simulink library "gbt_library"  (Simulink 7.4)
settings: Solver=ode45  StartTime=0.0  StopTime=10.0  RelTol=1e-3
undefined symbols (not defined in the file or in its folder): xlipgetpartsetting
libraries: xbsIndex_r4 x1348, casper_library_misc x29, casper_library_flow_control x4
(part 1 of 11)
settings Model: Creator=mwagner  LastModifiedBy=chenhong

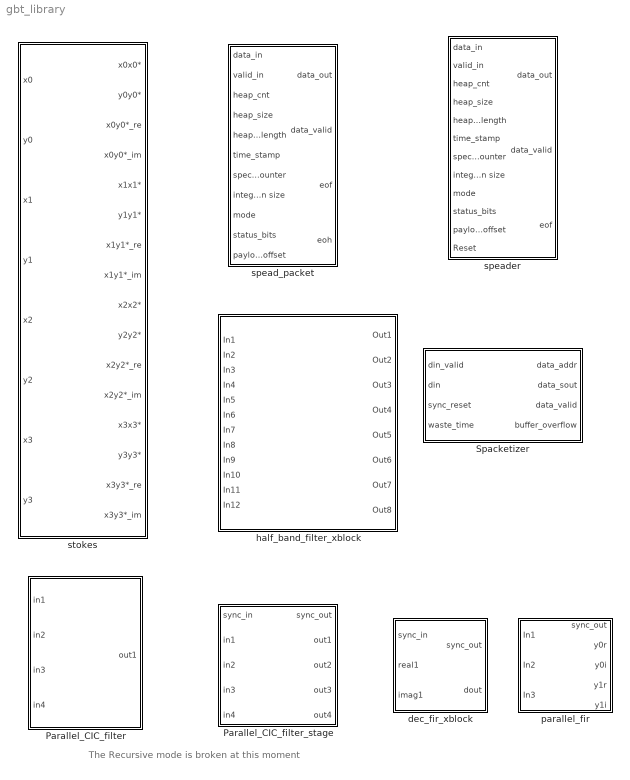
== system gbt_library ==
  note: The Recursive mode is broken at this moment
  Parallel_CIC_filter : Subsystem  mask(Parallel_CIC_filter){m=3, n=100, n_inputs=4, polyphase=off, add_latency=1, n_bits=8, bin_pt=7, dec2_halfout=on, half2first=off, recursive=off}
      mask prompts: m "CIC filter Order"; n "Decimation rate"; polyphase "polyphase structure?(Effective only when n_inputs = 1 or n_inputs = dec_rate)"; add_latency "Add latency"; n_bits "Input bit width"; bin_pt "Binary point"; dec2_halfout "When dec_rate =2, half the number of outputs?"; half2first "Order of stages: Smaller prime factors first?"; recursive "Recursive structure"
      mask help:
      | A non-recursive CIC filter with parallel inputs.
      | Decimation rate is factored into prime numbers. Each implemented using a single stage.
      |
      | For each stages:
      | Only supports decimation rate that is a prime number.
      | If dec_rate = 2, then n_outputs = 0.5*n_inputs.
      | In other cases, n_outputs = n_inputs.
      | Polyphase structure available for stages of n_inputs is 1 or 2.
      mask init:
      | config.source=str2func('parallel_cic_filter_init_xblock');
      | config.toplevel=gcb;
      | set_param(config.toplevel, 'LinkStatus','inactive');
      | xBlock(config, {m,n,n_inputs,...
      |                 polyphase,add_latency,...
      |                 dec2_halfout, half2first,...
      |                 n_bits, bin_pt, recursive} ...
      |                 );
  Parallel_CIC_filter_stage : Subsystem  mask(Parallel_CIC_filter_stage){m=3, n=7, n_inputs=4, polyphase=off, add_latency=1, n_bits=8, bin_pt=7, dec2_halfout=on, recursive=off}
      mask prompts: m "CIC filter Order"; n "Decimation rate"; polyphase "polyphase structure?(Effective only when n_inputs = 1 or n_inputs = dec_rate)"; add_latency "Add latency"; n_bits "Input bit width"; bin_pt "Binary point"; dec2_halfout "When dec_rate =2, half the number of outputs?"; recursive "Recursive structure?"
      mask help:
      | A single stage of CIC filter with parallel inputs.
      | Only supports decimation rate that is a prime number.
      | If dec_rate = 2, then n_outputs = 0.5*n_inputs.
      | In other cases, n_outputs = n_inputs.
      | Polyphase structure available when n_inputs is 1 or 2.
      mask init:
      | xBlock;
      | config.source=str2func('parallel_polynomial_dec_stage_init_xblock');
      | config.toplevel=gcb;
      | xBlock(config, {m,n,n_inputs, ...
      |                 polyphase,add_latency, ...
      |                 dec2_halfout, n_bits, bin_pt,recursive} ...
      |                 );
  Spacketizer : Subsystem  AncestorBlock=gbt_library/packetizer  mask(packetizer){pin_width=256, sout_width=64, fifo_depth=128, total_words=32}
      mask prompts: pin_width "Parallel Input Width"; sout_width "Serial Output Width"; fifo_depth "FIFO depth"; total_words "Total number of data points"
      mask help:
      | This block is intended to serialize data that is 'bursty', that is,
      | the average data rate is small but per cycle the data is highly
      | parallel and can contain many points simultaneously.  This situation
      | is common with the streaming CASPER FFTs and related blocks.
      |
      | The serialization buffers the data when valid and independently
      | serializes the data when the buffer is non-empty.  For convenience, the
      | data is counted as it is serialized and signals exist to indicate
      | that the serial output is valid or that a buffer overflow has occured.  The
      | block will not stop in the case of an overflow, and the overflow
      | signal is not held high after it occurs.
      |
      | For example usage, see 'roach_spec_2adc_borph' in 'SVNROOT/trunk/projects/roach_spec/'
      | or the test case in 'SVNROOT/trunk/mlib_devel_10_1/Tests/packetizer_test.mdl'
      |
      | For extended documentation, please see the CASPER wiki
      mask init:
      | packetizer_init(gcb, 'pin_width', pin_width, 'sout_width', sout_width, 'total_words', total_words, 'fifo_depth', fifo_depth)
      | % packetizer_init(gcb, ...
      | %     'pin_width', pin_width, ...
      | %     'sout_width', sout_width, ...
      | %   %  'fifo_depth', fifo_depth, ...
      | %     'total_words', total_words);
      settings: AttributesFormatString=|
      | Parallel Input Width: 256
      | Serial Output Width: 64
      mask StyleString: edit,edit,popup(16|32|64|128|256|512|1K|2K|4K|8K|16K|32K|64K),edit
  dec_fir_xblock : Subsystem  mask{n_inputs=1, coeff=[0 0], n_bits=4, quantization=Truncate, add_latency=1, mult_latency=2, coeff_bit_width=25, coeff_bin_pt=24, adder_tree_hdl=on}
      mask prompts: n_inputs "Number of Parallel Streams"; coeff "Coefficients"; n_bits "Bit Width Out"; quantization "Quantization Behavior"; add_latency "Add Latency"; mult_latency "Mult Latency"; coeff_bit_width "Coefficient bit width"; coeff_bin_pt "Coefficient binary point"; adder_tree_hdl "Implement first stage of adder trees after multiplication as behavioural HDL"
      mask init:
      | config.source=str2func('dec_fir_init_xblock');
      | config.toplevel=gcb;
      | xBlock(config, ...
      |         {n_inputs,coeff,n_bits,quantization,add_latency,...
      |          mult_latency, coeff_bit_width,coeff_bin_pt,adder_tree_hdl})
      mask StyleString: edit,edit,edit,popup(Truncate|Round  (unbiased: +/- Inf)|Round  (unbiased: Even Values)),edit,edit,edit,edit,checkbox
  half_band_filter_xblock : Subsystem  mask{filter_coeffs=4}
      mask prompts: filter_coeffs "Parallel FIR filter Coefficients"
      mask init:
      | config.source=str2func('half_band_init_xblock');
      | config.toplevel=gcb;
      | xBlock(config, ...
      |         {filter_coeffs})
  parallel_fir : Subsystem  mask(Parallel FIR Filter){filter_coeffs=4}
      mask prompts: filter_coeffs "Filter coefficients"
      mask help: Xblock
      mask init:
      | config.source=str2func('parallel_fir_init_xblock');
      | config.toplevel=gcb;
      | xBlock(config, ...
      |         {filter_coeffs})
  spead_packet : Subsystem  AncestorBlock=gbt_library/spead_packet  mask{spead_msw=64, spead_lsw=40, pkt_bits=6, fifo_latency=4}
      mask help: The size of the heap and payload are in Bytes. If there is one packet per heap then payload_offset is 0. All the input must be not longer than 40 bits.
  speader : Subsystem  AncestorBlock=gbt_library/spead_packet  mask{spead_msw=64, spead_lsw=40, num_items=6}
      mask prompts: num_items "Number of items (+5)"
      mask help:
      | The size of the heap and payload are in Bytes.
      | If there is one packet per heap then payload_offset is 0.
      | All the input must be not longer than 40 bits.
  stokes : Subsystem  mask{n_samples=4}
      mask prompts: n_samples "Number of Simultaneous Inputs"
      mask init:
      | % To make the xBlock smart so it won''t re-generate the
      | % subsystem if neither the arguments nor the scripts are
      | % changes, use as the following:
      | cfg.source = str2func('stokes_init');
      | cfg.toplevel = gcb;
      | cfg.depend = {'stokes_init'};
      | args = {n_samples};
      | xBlock(cfg, args);
      mask TabNameString: Basic

== system gbt_library/Parallel_CIC_filter ==
  in1 : Inport
  in2 : Inport  Port=2
  in3 : Inport  Port=3
  in4 : Inport  Port=4
  Stage1_dec5 : Subsystem
  Stage2_dec5 : Subsystem
  Stage3_dec2 : Subsystem
  Stage4_dec2 : Subsystem
  Terminator{1..4} (4 alike) : Terminator
  out1 : Outport
  wires:
  in1/1 -> Stage4_dec2/1(sync_in), Stage3_dec2/1(sync_in), Stage2_dec5/1(sync_in), Stage1_dec5/2(in1), Stage1_dec5/1(sync_in)
  Stage4_dec2/1(sync_out) -> Terminator4/1  "ter4"
  Stage3_dec2/1(sync_out) -> Terminator3/1  "ter3"
  Stage2_dec5/1(sync_out) -> Terminator2/1  "ter2"
  Stage1_dec5/1(sync_out) -> Terminator1/1  "ter1"
  Stage4_dec2/2(out1) -> out1/1
  Stage3_dec2/3(out2) -> Stage4_dec2/3(in2)  "sig4_2"
  Stage3_dec2/2(out1) -> Stage4_dec2/2(in1)  "sig4_1"
  Stage2_dec5/5(out4) -> Stage3_dec2/5(in4)  "sig3_4"
  Stage2_dec5/4(out3) -> Stage3_dec2/4(in3)  "sig3_3"
  Stage2_dec5/3(out2) -> Stage3_dec2/3(in2)  "sig3_2"
  Stage2_dec5/2(out1) -> Stage3_dec2/2(in1)  "sig3_1"
  Stage1_dec5/5(out4) -> Stage2_dec5/5(in4)  "sig2_4"
  Stage1_dec5/4(out3) -> Stage2_dec5/4(in3)  "sig2_3"
  Stage1_dec5/3(out2) -> Stage2_dec5/3(in2)  "sig2_2"
  Stage1_dec5/2(out1) -> Stage2_dec5/2(in1)  "sig2_1"
  in4/1 -> Stage1_dec5/5(in4)
  in3/1 -> Stage1_dec5/4(in3)
  in2/1 -> Stage1_dec5/3(in2)

== system gbt_library/Parallel_CIC_filter_stage ==
  sync_in : Inport
  in1 : Inport  Port=2
  in2 : Inport  Port=3
  in3 : Inport  Port=4
  in4 : Inport  Port=5
  decimator_7 : Subsystem
  p_adder1 : Subsystem
  p_adder2 : Subsystem
  p_adder3 : Subsystem
  sync_out : Outport
  out1 : Outport  Port=2
  out2 : Outport  Port=3
  out3 : Outport  Port=4
  out4 : Outport  Port=5
  wires:
  decimator_7/5(Out4) -> out4/1
  decimator_7/4(Out3) -> out3/1
  decimator_7/3(Out2) -> out2/1
  decimator_7/2(Out1) -> out1/1
  decimator_7/1(sync_out) -> sync_out/1
  p_adder3/5(out4) -> decimator_7/5(In4)  "pa_i4_4"
  p_adder3/4(out3) -> decimator_7/4(In3)  "pa_i4_3"
  p_adder3/3(out2) -> decimator_7/3(In2)  "pa_i4_2"
  p_adder3/2(out1) -> decimator_7/2(In1)  "pa_i4_1"
  p_adder3/1(sync_out) -> decimator_7/1(sync_in)  "sync_in4"
  p_adder2/5(out4) -> p_adder3/5(in4)  "pa_i3_4"
  p_adder2/4(out3) -> p_adder3/4(in3)  "pa_i3_3"
  p_adder2/3(out2) -> p_adder3/3(in2)  "pa_i3_2"
  p_adder2/2(out1) -> p_adder3/2(in1)  "pa_i3_1"
  p_adder2/1(sync_out) -> p_adder3/1(sync_in)  "sync_in3"
  p_adder1/5(out4) -> p_adder2/5(in4)  "pa_i2_4"
  p_adder1/4(out3) -> p_adder2/4(in3)  "pa_i2_3"
  p_adder1/3(out2) -> p_adder2/3(in2)  "pa_i2_2"
  p_adder1/2(out1) -> p_adder2/2(in1)  "pa_i2_1"
  p_adder1/1(sync_out) -> p_adder2/1(sync_in)  "sync_in2"
  in4/1 -> p_adder1/5(in4)
  in3/1 -> p_adder1/4(in3)
  in2/1 -> p_adder1/3(in2)
  in1/1 -> p_adder1/2(in1)
  sync_in/1 -> p_adder1/1(sync_in)

== system gbt_library/Spacketizer ==
  din_valid : Inport
  din : Inport  Port=2
  sync_reset : Inport  Port=3
  waste_time : Inport  Port=4
  Counter : xbsIndex_r4/Counter  cnt_type=Free Running  cnt_to=Inf  operation=Up  start_count=0  cnt_by_val=1  arith_type=Unsigned  n_bits=11  bin_pt=0  load_pin=off  rst=on  en=on  explicit_period=on  period=1  dbl_ovrd=off  use_behavioral_HDL=off  implementation=Fabric  use_rpm=off  block_type=counter
  Inverter : xbsIndex_r4/Inverter  en=off  latency=0  dbl_ovrd=off  block_type=inv
  Logical : xbsIndex_r4/Logical  logical_function=AND  inputs=2  en=off  latency=0  precision=Full  arith_type=Unsigned  n_bits=16  bin_pt=0  align_bp=on  dbl_ovrd=off  block_type=logical
  Logical1 : xbsIndex_r4/Logical  logical_function=AND  inputs=2  en=off  latency=0  precision=Full  arith_type=Unsigned  n_bits=16  bin_pt=0  align_bp=on  dbl_ovrd=off  block_type=logical
  data_buffer : xbsIndex_r4/FIFO  depth=128  percent_nbits=1  rst=off  en=off  use_dcount=off  use_almost_empty=off  almost_empty_thresh=2  use_almost_full=off  almost_full_thresh=14  dbl_ovrd=off  mem_type=Block RAM  explicit_period=off  block_type=fifo
      settings: block_version=10.1.3
  data_counter : xbsIndex_r4/Counter  cnt_type=Free Running  cnt_to=Inf  operation=Up  start_count=0  cnt_by_val=1  arith_type=Unsigned  n_bits=6  bin_pt=0  load_pin=off  rst=on  en=on  explicit_period=on  period=1  dbl_ovrd=off  use_behavioral_HDL=off  implementation=Fabric  use_rpm=off  block_type=counter
  packetizer_fsm : xbsIndex_r4/MCode  mfname=packetizer_fsm  explicit_period=off  period=1  inputsTable={'boundInpExpr'=>['','','3','','31','','',''],'inputs'=>['fifo_empty','shift_count','data_per_word','data_count','n_words','sync_reset','waste_count','waste_time']}  outputsTable={'outputs'=>['fifo_re','bram_addr_en','bram_we','serializer_shift','serializer_ld','shift_count_en','shift_count_rst','bram_addr_rst','data_count_en','data_count_rst','done','waste_count_en','waste_count_rst'],'suppressOut'=>['off','off','off','off','off','off','off','off','off','off','off','off','off']}  dbl_ovrd=off  enable_stdout=off  enable_debug=off  suppress_output=on  defparams={'data_per_word',3,'n_words',31}  hide_port_list={}  block_type=mcode
      settings: block_version=11.4
  parallel_to_serial_converter : Subsystem  AncestorBlock=casper_library/Flow_Control/parallel_to_serial_converter  mask(parallel_to_serial_converter){pin_width=256, sout_width=64}
      mask prompts: pin_width "Parallel Input Width"; sout_width "Serial Output Width"
      mask help:
      | This block takes as input a parallel bus of specified width.
      | When the load signal 'ld' is asserted, this data is broken into
      | pieces of width specified by the serial output width and
      | stored into different registers chained to form a shift register.
      | If the 'shift' input is subsequently asserted, the shift register
      | returns as output a new piece of data of width sout_width.  This data
      | is the next least significant piece of the original bus.  The converter
      | serializes SMALL ENDIAN.
      |
      | Note that the load operation automatically loads the least significant
      | bits into the register closest to the output, so the first 'shift'
      | assertion changes the data output from bits [sout_width-1:0] to
      | bits [2*sout_width-1:sout_width].
      mask init:
      | parallel_to_serial_converter_init(gcb, ...
      |     'pin_width', pin_width, ...
      |     'sout_width', sout_width);
  shift_counter : xbsIndex_r4/Counter  cnt_type=Free Running  cnt_to=Inf  operation=Up  start_count=0  cnt_by_val=1  arith_type=Unsigned  n_bits=3  bin_pt=0  load_pin=off  rst=on  en=on  explicit_period=on  period=1  dbl_ovrd=off  use_behavioral_HDL=off  implementation=Fabric  use_rpm=off  block_type=counter
  waste_counter : xbsIndex_r4/Counter  cnt_type=Free Running  cnt_to=Inf  operation=Up  start_count=0  cnt_by_val=1  arith_type=Unsigned  n_bits=5  bin_pt=0  load_pin=off  rst=on  en=on  explicit_period=on  period=1  dbl_ovrd=off  use_behavioral_HDL=off  implementation=Fabric  use_rpm=off  block_type=counter
  data_addr : Outport
  data_sout : Outport  Port=2
  data_valid : Outport  Port=3
  buffer_overflow : Outport  Port=4
  wires:
  waste_time/1 -> packetizer_fsm/6
  packetizer_fsm/13 -> waste_counter/1
  packetizer_fsm/12 -> waste_counter/2
  waste_counter/1 -> packetizer_fsm/5
  sync_reset/1 -> packetizer_fsm/4
  packetizer_fsm/10 -> data_counter/1
  data_counter/1 -> packetizer_fsm/3
  packetizer_fsm/9 -> data_counter/2
  packetizer_fsm/8 -> Counter/1
  packetizer_fsm/2 -> Counter/2
  Counter/1 -> data_addr/1
  data_buffer/2 -> packetizer_fsm/1
  packetizer_fsm/7 -> shift_counter/1
  shift_counter/1 -> packetizer_fsm/2
  packetizer_fsm/6 -> shift_counter/2
  parallel_to_serial_converter/1(sout) -> data_sout/1
  din/1 -> data_buffer/1
  packetizer_fsm/3 -> data_valid/1
  packetizer_fsm/5 -> parallel_to_serial_converter/2(ld)
  packetizer_fsm/4 -> parallel_to_serial_converter/3(shift)
  packetizer_fsm/1 -> data_buffer/3
  data_buffer/1 -> parallel_to_serial_converter/1(pin)
  Logical/1 -> data_buffer/2
  din_valid/1 -> Logical/1, Logical1/1
  Inverter/1 -> Logical/2
  data_buffer/4 -> Inverter/1, Logical1/2
  Logical1/1 -> buffer_overflow/1

== system gbt_library/dec_fir_xblock ==
  sync_in : Inport
  real1 : Inport  Port=2
  imag1 : Inport  Port=3
  convert1 : xbsIndex_r4/Convert  arith_type="Signed  (2's comp)"  n_bits=4  bin_pt=3  quantization=Truncate  overflow=Wrap  latency=1  dbl_ovrd=off  pipeline=off  block_type=convert
      settings: block_version=11.4
  convert2 : xbsIndex_r4/Convert  arith_type="Signed  (2's comp)"  n_bits=4  bin_pt=3  quantization=Truncate  overflow=Wrap  latency=1  dbl_ovrd=off  pipeline=off  block_type=convert
      settings: block_version=11.4
  delay : xbsIndex_r4/Delay  en=off  latency=4  dbl_ovrd=off  reg_retiming=off  block_type=delay
      settings: block_version=11.4
  fir_dbl_col1 : Subsystem
  imag_sum : Subsystem
  real_sum : Subsystem
  ri_to_c : casper_library_misc/ri_to_c  SystemSampleTime=-1
  shift1 : xbsIndex_r4/Shift  shift_dir=Left  shift_bits=1  en=off  latency=0  precision=Full  arith_type="Signed  (2's comp)"  n_bits=16  bin_pt=14  quantization=Truncate  overflow=Wrap  dbl_ovrd=off  block_type=shift
  shift2 : xbsIndex_r4/Shift  shift_dir=Left  shift_bits=1  en=off  latency=0  precision=Full  arith_type="Signed  (2's comp)"  n_bits=16  bin_pt=14  quantization=Truncate  overflow=Wrap  dbl_ovrd=off  block_type=shift
  sync_out : Outport
  dout : Outport  Port=2
  wires:
  delay/1 -> real_sum/1(sync), imag_sum/1(sync)
  shift2/1 -> convert2/1
  imag_sum/2(dout) -> shift2/1
  shift1/1 -> convert1/1
  real_sum/2(dout) -> shift1/1
  ri_to_c/1 -> dout/1
  convert2/1 -> ri_to_c/2
  convert1/1 -> ri_to_c/1
  real_sum/1(sync_out) -> sync_out/1
  fir_dbl_col1/5(real_sum) -> real_sum/2(din_1)  "xlsub2_fir_col1_5"
  fir_dbl_col1/6(imag_sum) -> imag_sum/2(din_1)  "xlsub2_fir_col1_6"
  fir_dbl_col1/2(imag_out1) -> fir_dbl_col1/4(imag_back1)  "xlsub2_fir_col1_2"
  fir_dbl_col1/1(real_out1) -> fir_dbl_col1/3(real_back1)  "xlsub2_fir_col1_1"
  imag1/1 -> fir_dbl_col1/2(imag1)
  real1/1 -> fir_dbl_col1/1(real1)
  sync_in/1 -> delay/1

== system gbt_library/half_band_filter_xblock ==
  In1 : Inport
  In2 : Inport  Port=2
  In3 : Inport  Port=3
  In4 : Inport  Port=4
  In5 : Inport  Port=5
  In6 : Inport  Port=6
  In7 : Inport  Port=7
  In8 : Inport  Port=8
  In9 : Inport  Port=9
  In10 : Inport  Port=10
  In11 : Inport  Port=11
  In12 : Inport  Port=12
  adder_tree : Subsystem
  adder_tree1 : Subsystem
  adder_tree3 : Subsystem
  adder_tree4 : Subsystem
  parallel_fir : Subsystem
  parallel_fir1 : Subsystem
  parallel_fir2 : Subsystem
  parallel_fir3 : Subsystem
  Out1 : Outport
  Out2 : Outport  Port=2
  Out3 : Outport  Port=3
  Out4 : Outport  Port=4
  Out5 : Outport  Port=5
  Out6 : Outport  Port=6
  Out7 : Outport  Port=7
  Out8 : Outport  Port=8
  wires:
  parallel_fir3/5(y1i) -> adder_tree4/5(din_4)
  parallel_fir3/4(y1r) -> adder_tree3/5(din_4)
  parallel_fir3/3(y0i) -> adder_tree1/5(din_4)
  parallel_fir3/2(y0r) -> adder_tree/5(din_4)
  parallel_fir3/1(sync_out) -> adder_tree4/1(sync)
  In12/1 -> parallel_fir3/3(In3)
  In11/1 -> parallel_fir3/2(In2)
  In10/1 -> parallel_fir3/1(In1)
  parallel_fir2/5(y1i) -> adder_tree4/4(din_3)
  parallel_fir2/4(y1r) -> adder_tree3/4(din_3)
  parallel_fir2/3(y0i) -> adder_tree1/4(din_3)
  parallel_fir2/2(y0r) -> adder_tree/4(din_3)
  parallel_fir2/1(sync_out) -> adder_tree3/1(sync)
  In9/1 -> parallel_fir2/3(In3)
  In8/1 -> parallel_fir2/2(In2)
  In7/1 -> parallel_fir2/1(In1)
  parallel_fir1/5(y1i) -> adder_tree4/3(din_2)
  parallel_fir1/4(y1r) -> adder_tree3/3(din_2)
  parallel_fir1/3(y0i) -> adder_tree1/3(din_2)
  parallel_fir1/2(y0r) -> adder_tree/3(din_2)
  parallel_fir1/1(sync_out) -> adder_tree1/1(sync)
  In6/1 -> parallel_fir1/3(In3)
  In5/1 -> parallel_fir1/2(In2)
  In4/1 -> parallel_fir1/1(In1)
  parallel_fir/5(y1i) -> adder_tree4/2(din_1)
  parallel_fir/4(y1r) -> adder_tree3/2(din_1)
  parallel_fir/3(y0i) -> adder_tree1/2(din_1)
  parallel_fir/2(y0r) -> adder_tree/2(din_1)
  parallel_fir/1(sync_out) -> adder_tree/1(sync)
  In3/1 -> parallel_fir/3(In3)
  In2/1 -> parallel_fir/2(In2)
  In1/1 -> parallel_fir/1(In1)
  adder_tree4/2(dout) -> Out8/1
  adder_tree4/1(sync_out) -> Out7/1
  adder_tree3/2(dout) -> Out6/1
  adder_tree3/1(sync_out) -> Out5/1
  adder_tree1/2(dout) -> Out4/1
  adder_tree1/1(sync_out) -> Out3/1
  adder_tree/2(dout) -> Out2/1
  adder_tree/1(sync_out) -> Out1/1

== system gbt_library/parallel_fir ==
  In1 : Inport
  In2 : Inport  Port=2
  In3 : Inport  Port=3
  AddSub{1,3,5..6} (4 alike) : xbsIndex_r4/AddSub  mode=Subtraction  use_carryin=off  use_carryout=off  en=off  latency=0  precision=Full  arith_type=Unsigned  n_bits=16  bin_pt=14  quantization=Truncate  overflow=Wrap  dbl_ovrd=off  use_behavioral_HDL=off  hw_selection=Fabric  pipelined=off  block_type=addsub
  AddSub2 : xbsIndex_r4/AddSub  mode=Addition  use_carryin=off  use_carryout=off  en=off  latency=0  precision=Full  arith_type=Unsigned  n_bits=16  bin_pt=14  quantization=Truncate  overflow=Wrap  dbl_ovrd=off  use_behavioral_HDL=off  hw_selection=Fabric  pipelined=off  block_type=addsub
  AddSub4 : xbsIndex_r4/AddSub  mode=Addition  use_carryin=off  use_carryout=off  en=off  latency=0  precision=Full  arith_type=Unsigned  n_bits=16  bin_pt=14  quantization=Truncate  overflow=Wrap  dbl_ovrd=off  use_behavioral_HDL=off  hw_selection=Fabric  pipelined=off  block_type=addsub
  Delay : xbsIndex_r4/Delay  en=off  latency=1  dbl_ovrd=off  reg_retiming=off  block_type=delay
      settings: block_version=11.4
  Delay1 : xbsIndex_r4/Delay  en=off  latency=1  dbl_ovrd=off  reg_retiming=off  block_type=delay
      settings: block_version=11.4
  c_to_ri : Subsystem
  c_to_ri1 : Subsystem
  c_to_ri2 : Subsystem
  f0 : Subsystem
  f0pf1 : Subsystem
  f1 : Subsystem
  sync_out : Outport
  y0r : Outport  Port=2
  y0i : Outport  Port=3
  y1r : Outport  Port=4
  y1i : Outport  Port=5
  wires:
  c_to_ri/1(re) -> AddSub5/1, AddSub2/1
  c_to_ri/2(im) -> AddSub6/1, AddSub4/1
  c_to_ri2/1(re) -> Delay/1, AddSub1/2
  c_to_ri2/2(im) -> Delay1/1, AddSub3/2
  In1/1 -> f1/1(sync_in), f0pf1/1(sync_in), f0/1(sync_in)
  In2/1 -> f1/2(real1), f0pf1/2(real1), f0/2(real1)
  In3/1 -> f1/3(imag1), f0pf1/3(imag1), f0/3(imag1)
  f1/2(dout) -> c_to_ri2/1(c)
  f0pf1/2(dout) -> c_to_ri1/1(c)
  f0/2(dout) -> c_to_ri/1(c)
  f0/1(sync_out) -> sync_out/1
  c_to_ri1/2(im) -> AddSub3/1
  c_to_ri1/1(re) -> AddSub1/1
  Delay1/1 -> AddSub4/2
  Delay/1 -> AddSub2/2
  AddSub6/1 -> y1i/1
  AddSub3/1 -> AddSub6/2
  AddSub5/1 -> y1r/1
  AddSub1/1 -> AddSub5/2
  AddSub4/1 -> y0i/1
  AddSub2/1 -> y0r/1

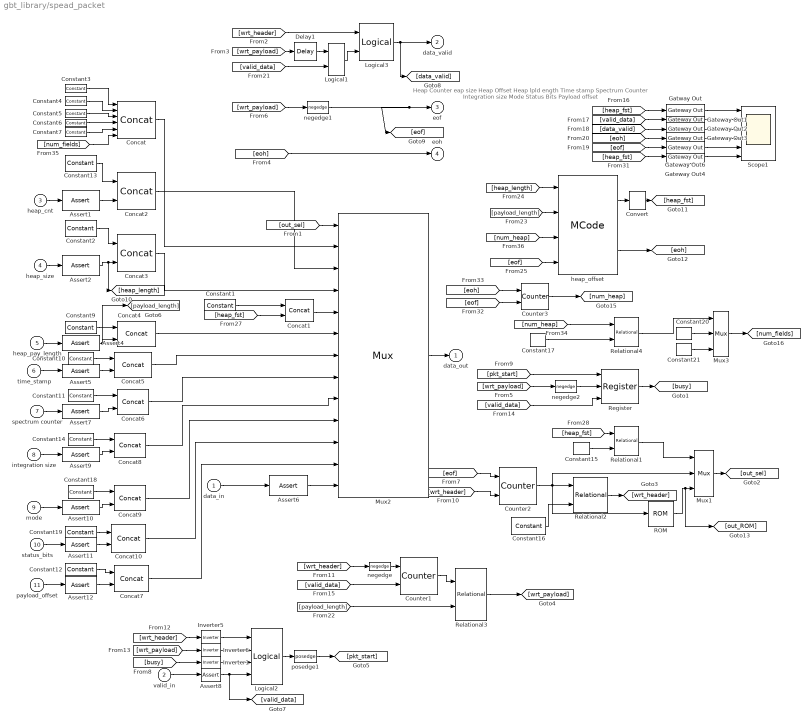
== system gbt_library/spead_packet ==
  note: Heap Counter
      | eap size
      | Heap Offset
      | Heap lpld ength
      | Time stamp
      | Spectrum Counter
      | Integration size
      | Mode
      | Status Bits
      | Payload offset
  data_in : Inport
  valid_in : Inport  Port=2
  heap_cnt : Inport  Port=3
  heap_size : Inport  Port=4
  heap_pay_length : Inport  Port=5
  time_stamp : Inport  Port=6
  spectrum counter : Inport  Port=7
  integration size : Inport  Port=8
  mode : Inport  Port=9
  status_bits : Inport  Port=10
  payload_offset : Inport  Port=11
  Assert{1..2,4..5,7,9..12} (9 alike) : xbsIndex_r4/Assert  assert_type=on  type_source=Explicitly  arith_type=Unsigned  n_bits=spead_lsw  bin_pt=0  assert_rate=off  rate_source=Explicitly  period=1  output_port=on  block_type=assert
      settings: block_version=11.4
  Assert6 : xbsIndex_r4/Assert  assert_type=on  type_source=Explicitly  arith_type=Unsigned  n_bits=64  bin_pt=0  assert_rate=off  rate_source=Explicitly  period=1  output_port=on  block_type=assert
      settings: block_version=11.4
  Assert8 : xbsIndex_r4/Assert  assert_type=on  type_source=Explicitly  arith_type=Boolean  n_bits=64  bin_pt=0  assert_rate=off  rate_source=Explicitly  period=1  output_port=on  block_type=assert
      settings: block_version=11.4
  Concat : xbsIndex_r4/Concat  num_inputs=6  dbl_ovrd=off  block_type=concat
  Concat{1..10} (10 alike) : xbsIndex_r4/Concat  num_inputs=2  dbl_ovrd=off  block_type=concat
  Constant1 : xbsIndex_r4/Constant  arith_type=Unsigned  const=8388611  n_bits=spead_msw-spead_lsw  bin_pt=0  explicit_period=on  period=1  equ=P=C  opselect=C  inp2=PCIN>>17  opr=+  inp1=P  carry=CIN  dbl_ovrd=off  block_type=constant
      settings: block_version=11.4
  Constant10 : xbsIndex_r4/Constant  arith_type=Unsigned  const=8388628  n_bits=spead_msw-spead_lsw  bin_pt=0  explicit_period=on  period=1  equ=P=C  opselect=C  inp2=PCIN>>17  opr=+  inp1=P  carry=CIN  dbl_ovrd=off  block_type=constant
      settings: block_version=11.4
  Constant11 : xbsIndex_r4/Constant  arith_type=Unsigned  const=8388629  n_bits=spead_msw-spead_lsw  bin_pt=0  explicit_period=on  period=1  equ=P=C  opselect=C  inp2=PCIN>>17  opr=+  inp1=P  carry=CIN  dbl_ovrd=off  block_type=constant
      settings: block_version=11.4
  Constant12 : xbsIndex_r4/Constant  arith_type=Unsigned  const=26  n_bits=spead_msw-spead_lsw  bin_pt=0  explicit_period=on  period=1  equ=P=C  opselect=C  inp2=PCIN>>17  opr=+  inp1=P  carry=CIN  dbl_ovrd=off  block_type=constant
      settings: block_version=11.4
  Constant13 : xbsIndex_r4/Constant  arith_type=Unsigned  const=8388609  n_bits=spead_msw-spead_lsw  bin_pt=0  explicit_period=on  period=1  equ=P=C  opselect=C  inp2=PCIN>>17  opr=+  inp1=P  carry=CIN  dbl_ovrd=off  block_type=constant
      settings: block_version=11.4
  Constant14 : xbsIndex_r4/Constant  arith_type=Unsigned  const=8388630  n_bits=spead_msw-spead_lsw  bin_pt=0  explicit_period=on  period=1  equ=P=C  opselect=C  inp2=PCIN>>17  opr=+  inp1=P  carry=CIN  dbl_ovrd=off  block_type=constant
      settings: block_version=11.4
  Constant15 : xbsIndex_r4/Constant  arith_type=Unsigned  const=0  n_bits=4  bin_pt=0  explicit_period=on  period=1  equ=P=C  opselect=C  inp2=PCIN>>17  opr=+  inp1=P  carry=CIN  dbl_ovrd=off  block_type=constant
      settings: block_version=11.4
  Constant16 : xbsIndex_r4/Constant  arith_type=Unsigned  const=11  n_bits=4  bin_pt=0  explicit_period=on  period=1  equ=P=C  opselect=C  inp2=PCIN>>17  opr=+  inp1=P  carry=CIN  dbl_ovrd=off  block_type=constant
      settings: block_version=11.4
  Constant17 : xbsIndex_r4/Constant  arith_type=Unsigned  const=0  n_bits=4  bin_pt=0  explicit_period=on  period=1  equ=P=C  opselect=C  inp2=PCIN>>17  opr=+  inp1=P  carry=CIN  dbl_ovrd=off  block_type=constant
      settings: block_version=11.4
  Constant18 : xbsIndex_r4/Constant  arith_type=Unsigned  const=8388631  n_bits=spead_msw-spead_lsw  bin_pt=0  explicit_period=on  period=1  equ=P=C  opselect=C  inp2=PCIN>>17  opr=+  inp1=P  carry=CIN  dbl_ovrd=off  block_type=constant
      settings: block_version=11.4
  Constant19 : xbsIndex_r4/Constant  arith_type=Unsigned  const=8388632  n_bits=spead_msw-spead_lsw  bin_pt=0  explicit_period=on  period=1  equ=P=C  opselect=C  inp2=PCIN>>17  opr=+  inp1=P  carry=CIN  dbl_ovrd=off  block_type=constant
      settings: block_version=11.4
  Constant2 : xbsIndex_r4/Constant  arith_type=Unsigned  const=8388610  n_bits=spead_msw-spead_lsw  bin_pt=0  explicit_period=on  period=1  equ=P=C  opselect=C  inp2=PCIN>>17  opr=+  inp1=P  carry=CIN  dbl_ovrd=off  block_type=constant
      settings: block_version=11.4
  Constant20 : xbsIndex_r4/Constant  arith_type=Unsigned  const=11  n_bits=8  bin_pt=0  explicit_period=on  period=1  equ=P=C  opselect=C  inp2=PCIN>>17  opr=+  inp1=P  carry=CIN  dbl_ovrd=off  block_type=constant
      settings: block_version=11.4
  Constant21 : xbsIndex_r4/Constant  arith_type=Unsigned  const=4  n_bits=8  bin_pt=0  explicit_period=on  period=1  equ=P=C  opselect=C  inp2=PCIN>>17  opr=+  inp1=P  carry=CIN  dbl_ovrd=off  block_type=constant
      settings: block_version=11.4
  Constant3 : xbsIndex_r4/Constant  arith_type=Unsigned  const=83  n_bits=8  bin_pt=0  explicit_period=on  period=1  equ=P=C  opselect=C  inp2=PCIN>>17  opr=+  inp1=P  carry=CIN  dbl_ovrd=off  block_type=constant
      settings: block_version=11.4
  Constant4 : xbsIndex_r4/Constant  arith_type=Unsigned  const=4  n_bits=8  bin_pt=0  explicit_period=on  period=1  equ=P=C  opselect=C  inp2=PCIN>>17  opr=+  inp1=P  carry=CIN  dbl_ovrd=off  block_type=constant
      settings: block_version=11.4
  Constant5 : xbsIndex_r4/Constant  arith_type=Unsigned  const=3  n_bits=8  bin_pt=0  explicit_period=on  period=1  equ=P=C  opselect=C  inp2=PCIN>>17  opr=+  inp1=P  carry=CIN  dbl_ovrd=off  block_type=constant
      settings: block_version=11.4
  Constant6 : xbsIndex_r4/Constant  arith_type=Unsigned  const=5  n_bits=8  bin_pt=0  explicit_period=on  period=1  equ=P=C  opselect=C  inp2=PCIN>>17  opr=+  inp1=P  carry=CIN  dbl_ovrd=off  block_type=constant
      settings: block_version=11.4
  Constant7 : xbsIndex_r4/Constant  arith_type=Unsigned  const=0  n_bits=16  bin_pt=0  explicit_period=on  period=1  equ=P=C  opselect=C  inp2=PCIN>>17  opr=+  inp1=P  carry=CIN  dbl_ovrd=off  block_type=constant
      settings: block_version=11.4
  Constant9 : xbsIndex_r4/Constant  arith_type=Unsigned  const=8388612  n_bits=spead_msw-spead_lsw  bin_pt=0  explicit_period=on  period=1  equ=P=C  opselect=C  inp2=PCIN>>17  opr=+  inp1=P  carry=CIN  dbl_ovrd=off  block_type=constant
      settings: block_version=11.4
  Convert : xbsIndex_r4/Convert  arith_type=Unsigned  n_bits=40  bin_pt=0  quantization=Truncate  overflow=Wrap  latency=0  dbl_ovrd=off  pipeline=off  block_type=convert
      settings: block_version=11.4
  Counter1 : xbsIndex_r4/Counter  cnt_type=Free Running  cnt_to=1023  operation=Up  start_count=0  cnt_by_val=1  arith_type=Unsigned  n_bits=pkt_bits+1  bin_pt=0  load_pin=off  rst=on  en=on  explicit_period=on  period=1  dbl_ovrd=off  use_behavioral_HDL=off  implementation=Fabric  use_rpm=on  block_type=counter
      settings: block_version=11.4
  Counter2 : xbsIndex_r4/Counter  cnt_type=Free Running  cnt_to=1023  operation=Up  start_count=0  cnt_by_val=1  arith_type=Unsigned  n_bits=4  bin_pt=0  load_pin=off  rst=on  en=on  explicit_period=on  period=1  dbl_ovrd=off  use_behavioral_HDL=off  implementation=Fabric  use_rpm=on  block_type=counter
      settings: block_version=11.4
  Counter3 : xbsIndex_r4/Counter  cnt_type=Free Running  cnt_to=1023  operation=Up  start_count=0  cnt_by_val=1  arith_type=Unsigned  n_bits=8  bin_pt=0  load_pin=off  rst=on  en=on  explicit_period=on  period=1  dbl_ovrd=off  use_behavioral_HDL=off  implementation=Fabric  use_rpm=on  block_type=counter
      settings: block_version=11.4
  Delay1 : xbsIndex_r4/Delay  en=off  latency=0  dbl_ovrd=off  reg_retiming=on  block_type=delay
      settings: block_version=11.4
  Gateway Out{1..4,6} (5 alike) : xbsIndex_r4/Gateway Out  hdl_port=on  timing_constraint=None  locs_specified=off  LOCs={}  block_type=gatewayout
      settings: infoedit="Gateway out block.  Converts Xilinx fixed point inputs into ouputs of type Simulink integer, double, or fixed point.<br><br>Hardware notes:  In hardware these blocks become top level output ports or are discarded, depending on how they are configured."  block_version=11.4
  Gatway Out : xbsIndex_r4/Gateway Out  hdl_port=on  timing_constraint=None  locs_specified=off  LOCs={}  block_type=gatewayout
      settings: infoedit="Gateway out block.  Converts Xilinx fixed point inputs into ouputs of type Simulink integer, double, or fixed point.<br><br>Hardware notes:  In hardware these blocks become top level output ports or are discarded, depending on how they are configured."  block_version=11.4
  Inverter1 : xbsIndex_r4/Inverter  en=off  latency=1  dbl_ovrd=off  block_type=inv
      settings: block_version=11.4
  Inverter5 : xbsIndex_r4/Inverter  en=off  latency=1  dbl_ovrd=off  block_type=inv
      settings: block_version=11.4
  Inverter6 : xbsIndex_r4/Inverter  en=off  latency=0  dbl_ovrd=off  block_type=inv
      settings: block_version=11.4
  Logical1 : xbsIndex_r4/Logical  logical_function=AND  inputs=2  en=off  latency=0  precision=Full  arith_type=Unsigned  n_bits=8  bin_pt=2  align_bp=on  dbl_ovrd=off  block_type=logical
      settings: block_version=11.4
  Logical2 : xbsIndex_r4/Logical  logical_function=AND  inputs=4  en=off  latency=0  precision=Full  arith_type=Unsigned  n_bits=8  bin_pt=2  align_bp=on  dbl_ovrd=off  block_type=logical
      settings: block_version=11.4
  Logical3 : xbsIndex_r4/Logical  logical_function=OR  inputs=2  en=off  latency=0  precision=Full  arith_type=Unsigned  n_bits=8  bin_pt=2  align_bp=on  dbl_ovrd=off  block_type=logical
      settings: block_version=11.4
  Mux1 : xbsIndex_r4/Mux  inputs=2  en=off  latency=0  precision=Full  arith_type="Signed  (2's comp)"  n_bits=8  bin_pt=2  quantization=Truncate  overflow=Wrap  dbl_ovrd=off  block_type=mux
      settings: block_version=11.4
  Mux2 : xbsIndex_r4/Mux  inputs=12  en=off  latency=0  precision=Full  arith_type="Signed  (2's comp)"  n_bits=8  bin_pt=2  quantization=Truncate  overflow=Wrap  dbl_ovrd=off  block_type=mux
      settings: block_version=11.4
  Mux3 : xbsIndex_r4/Mux  inputs=2  en=off  latency=0  precision=Full  arith_type="Signed  (2's comp)"  n_bits=8  bin_pt=2  quantization=Truncate  overflow=Wrap  dbl_ovrd=off  block_type=mux
      settings: block_version=11.4
  ROM : xbsIndex_r4/ROM  depth=12  initVector=[0 1 2 3 4 11 11 11 11 11 11 11]  distributed_mem=Distributed memory  rst=off  init_reg=0  en=off  latency=0  arith_type=Unsigned  n_bits=4  bin_pt=0  dbl_ovrd=off  optimize=Area  use_rpm=on  block_type=sprom
      settings: block_version=11.4
  Register : xbsIndex_r4/Register  init=0  rst=on  en=on  dbl_ovrd=off  block_type=register
      settings: block_version=11.4
  Relational1 : xbsIndex_r4/Relational  mode=a!=b  en=off  latency=0  dbl_ovrd=off  block_type=relational
  Relational2 : xbsIndex_r4/Relational  mode=a<b  en=off  latency=0  dbl_ovrd=off  block_type=relational
  Relational3 : xbsIndex_r4/Relational  mode=a<=b  en=off  latency=0  dbl_ovrd=off  block_type=relational
  Relational4 : xbsIndex_r4/Relational  mode=a>b  en=off  latency=0  dbl_ovrd=off  block_type=relational
  Scope1 : Scope  NumInputPorts=6
      settings: YMin=-5~-5~-5~-5~-5~-5  YMax=5~5~5~5~5~5  SaveName=ScopeData2  MaxDataPoints=10000
  heap_offset : xbsIndex_r4/MCode  mfname=heap_offset  explicit_period=off  period=1  inputsTable={'boundInpExpr'=>['','','',''],'inputs'=>['heap_length','pld_length','num_heap','eof']}  outputsTable={'outputs'=>['heap_offset_out','eoh'],'suppressOut'=>['off','off']}  dbl_ovrd=off  enable_stdout=off  enable_debug=off  suppress_output=on  defparams={}  hide_port_list={}  block_type=mcode
      settings: block_version=11.4
  negedge : casper_library_misc/negedge  Tag=Rising Edge Detector  SystemSampleTime=-1
  negedge1 : casper_library_misc/negedge  Tag=Rising Edge Detector  SystemSampleTime=-1
  negedge2 : casper_library_misc/negedge  Tag=Rising Edge Detector  SystemSampleTime=-1
  posedge1 : casper_library_misc/posedge  Tag=Rising Edge Detector  SystemSampleTime=-1
  data_out : Outport
  data_valid : Outport  Port=2
  eof : Outport  Port=3
  eoh : Outport  Port=4
  wires:
  Gateway Out3/1 -> Scope1/4
  Gateway Out6/1 -> Scope1/5
  Gateway Out4/1 -> Scope1/6
  Gateway Out2/1 -> Scope1/3
  Gateway Out1/1 -> Scope1/2
  Gatway Out/1 -> Scope1/1
  [num_heap] -> heap_offset/3
  [eof] -> heap_offset/4
  Mux3/1 -> [num_fields]
  Constant21/1 -> Mux3/3
  Constant20/1 -> Mux3/2
  Relational4/1 -> Mux3/1
  Constant17/1 -> Relational4/2
  [num_heap] -> Relational4/1
  Counter3/1 -> [num_heap]
  [eoh] -> Counter3/1
  [eof] -> Counter3/2
  [heap_fst] -> Gateway Out4/1
  Relational1/1 -> Mux1/1
  [heap_fst] -> Relational1/1
  Constant15/1 -> Relational1/2
  ROM/1 -> [out_ROM], Mux1/3
  Mux1/1 -> [out_sel]
  heap_offset/1 -> Convert/1
  Convert/1 -> [heap_fst]
  heap_offset/2 -> [eoh]
  [heap_fst] -> Concat1/2
  [heap_length] -> heap_offset/1
  [payload_length] -> heap_offset/2
  Constant16/1 -> Relational2/2
  Counter2/1 -> ROM/1, Mux1/2, Relational2/1
  Relational2/1 -> [wrt_header]
  [eof] -> Counter2/1
  [wrt_header] -> Counter2/2
  Relational3/1 -> [wrt_payload]
  Concat8/1 -> Mux2/9
  Constant14/1 -> Concat8/1
  Assert9/1 -> Concat8/2
  integration size/1 -> Assert9/1
  Concat5/1 -> Mux2/7
  Concat6/1 -> Mux2/8
  Constant11/1 -> Concat6/1
  Assert7/1 -> Concat6/2
  spectrum counter/1 -> Assert7/1
  Concat9/1 -> Mux2/10
  Concat10/1 -> Mux2/11
  Concat7/1 -> Mux2/12
  Assert6/1 -> Mux2/13
  Concat1/1 -> Mux2/5
  Constant1/1 -> Concat1/1
  [payload_length] -> Relational3/2
  [eof] -> Gateway Out6/1
  [valid_data] -> Logical1/2
  Logical1/1 -> Logical3/2
  Delay1/1 -> Logical1/1
  [eoh] -> Gateway Out3/1
  [data_valid] -> Gateway Out2/1
  [valid_data] -> Gateway Out1/1
  [heap_fst] -> Gatway Out/1
  [valid_data] -> Counter1/2
  [valid_data] -> Register/3
  heap_pay_length/1 -> Assert4/1
  Inverter5/1 -> Logical2/1
  [wrt_payload] -> Inverter6/1
  [wrt_header] -> Inverter5/1
  [wrt_header] -> negedge/1
  posedge1/1 -> [pkt_start]
  [pkt_start] -> Register/1
  [busy] -> Inverter1/1
  Register/1 -> [busy]
  [wrt_payload] -> negedge2/1
  [wrt_payload] -> negedge1/1
  [eoh] -> eoh/1
  [wrt_payload] -> Delay1/1
  [wrt_header] -> Logical3/1
  [out_sel] -> Mux2/1
  negedge1/1 -> [eof], eof/1
  Counter1/1 -> Relational3/1
  Mux2/1 -> data_out/1
  Concat2/1 -> Mux2/3
  Logical3/1 -> [data_valid], data_valid/1
  Inverter1/1 -> Logical2/3
  Assert5/1 -> Concat5/2
  Assert4/1 -> [payload_length], Concat4/2
  Assert2/1 -> [heap_length], Concat3/2
  Assert1/1 -> Concat2/2
  heap_cnt/1 -> Assert1/1
  heap_size/1 -> Assert2/1
  time_stamp/1 -> Assert5/1
  data_in/1 -> Assert6/1
  valid_in/1 -> Assert8/1
  Constant10/1 -> Concat5/1
  Constant12/1 -> Concat7/1
  Constant13/1 -> Concat2/1
  Constant2/1 -> Concat3/1
  Constant3/1 -> Concat/1
  Constant4/1 -> Concat/2
  Constant5/1 -> Concat/3
  Constant6/1 -> Concat/4
  Constant7/1 -> Concat/5
  [num_fields] -> Concat/6
  Constant9/1 -> Concat4/1
  Inverter6/1 -> Logical2/2
  Assert8/1 -> Logical2/4, [valid_data]
  Concat/1 -> Mux2/2
  Concat3/1 -> Mux2/4
  Concat4/1 -> Mux2/6
  negedge/1 -> Counter1/1
  negedge2/1 -> Register/2
  Logical2/1 -> posedge1/1
  Constant18/1 -> Concat9/1
  mode/1 -> Assert10/1
  Assert10/1 -> Concat9/2
  Constant19/1 -> Concat10/1
  status_bits/1 -> Assert11/1
  Assert11/1 -> Concat10/2
  payload_offset/1 -> Assert12/1
  Assert12/1 -> Concat7/2
